simulink model "QAM64_06"  (Simulink 6.6)
settings: Solver=VariableStepDiscrete  StartTime=0.0  StopTime=64*1024/112e6  RelTol=1e-3
undefined symbols (not defined in the file): get, xlfda_numerator
libraries: xbsIndex_r4 x20, dspsnks4 x4, dspsigops x2
settings Model: Creator=lcrockett  LastModifiedBy=lcrockett
settings OptimizationCC: InlineParams=on  InlineInvariantSignals=on
settings DebuggingCC: SignalResolutionControl=TryResolveAllWithWarning  MultiTaskDSMMsg=warning  MultiTaskCondExecSysMsg=none  StrictBusMsg=None
settings RTWCC: IncludeERTFirstTime=on

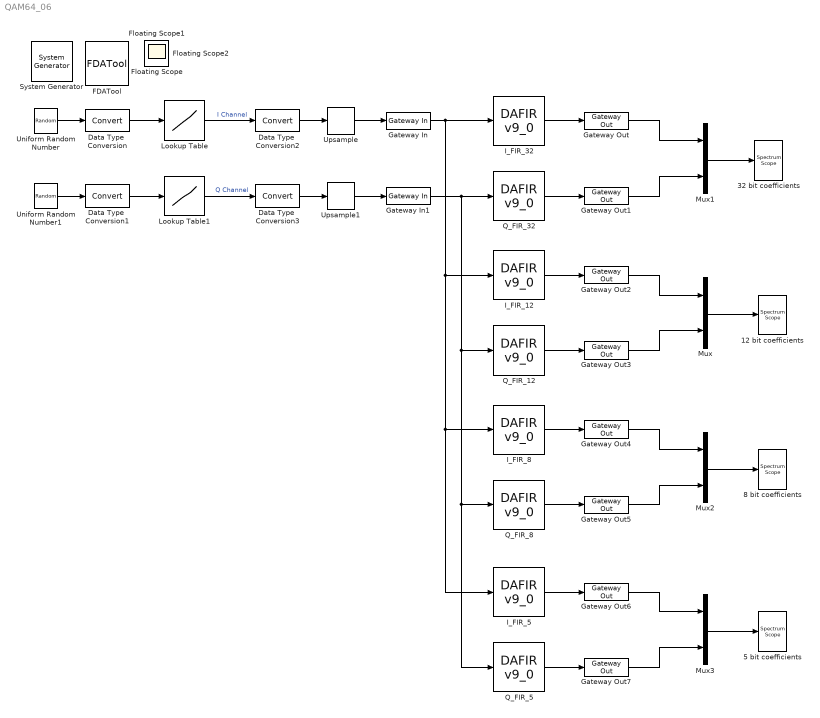
== system QAM64_06 ==
  " System Generator" : xbsIndex_r4/ System Generator  Tag=genX  SystemSampleTime=-1  xilinxfamily=Virtex2  part=xc2v1000  speed=-4  package=bg575  synthesis_tool=XST  directory=./netlist  testbench=off  simulink_period=1/112e6  sysclk_period=100  incr_netlist=off  trim_vbits=Everywhere in SubSystem  dbl_ovrd=According to Block Masks  core_generation=According to Block Masks  run_coregen=off  deprecated_control=off  eval_field=0  block_type=sysgen
      settings: block_version=9.2.01
  12 bit coefficients : dspsnks4/Spectrum Scope  DialogController=dspdialog.SpectrumScope  DialogControllerArgs=DataTag1  SystemSampleTime=-1  ScopeProperties=on  Domain=Frequency  HorizSpan=1  UseBuffer=on  BufferSize=1024  Overlap=64  inpFftLenInherit=on  FFTlength=1024  numAvg=2  DisplayProperties=off  AxisGrid=on  Memory=off  FrameNumber=on  AxisLegend=off  AxisZoom=off  OpenScopeAtSimStart=on  OpenScopeImmediately=off  FigPos=get(0,'defaultfigureposition')  AxisProperties=off  XUnits=Hertz  XRange=[0...Fs/2]  InheritXIncr=off  XIncr=1/112e6  XLabel=Samples  XLimit=Auto  YUnits=dB  XMax=1  XMin=0  YLabel=Magnitude, dB  LineProperties=off  LineColors=[1 0 0]|[0 0 1]  wintypeSpecScope=Hann  RsSpecScope=50  betaSpecScope=5  winsampSpecScope=Periodic
      settings: YMin=-70.9421156820398  YMax=37.379435684992
  32 bit coefficients : dspsnks4/Spectrum Scope  DialogController=dspdialog.SpectrumScope  DialogControllerArgs=DataTag2  SystemSampleTime=-1  ScopeProperties=on  Domain=Frequency  HorizSpan=1  UseBuffer=on  BufferSize=1024  Overlap=64  inpFftLenInherit=on  FFTlength=1024  numAvg=2  DisplayProperties=off  AxisGrid=on  Memory=off  FrameNumber=on  AxisLegend=off  AxisZoom=off  OpenScopeAtSimStart=on  OpenScopeImmediately=off  FigPos=get(0,'defaultfigureposition')  AxisProperties=off  XUnits=Hertz  XRange=[0...Fs/2]  InheritXIncr=off  XIncr=1/112e6  XLabel=Samples  XLimit=Auto  YUnits=dB  XMax=1  XMin=0  YLabel=Magnitude, dB  LineProperties=off  LineColors=[1 0 0]|[0 0 1]  wintypeSpecScope=Hann  RsSpecScope=50  betaSpecScope=5  winsampSpecScope=Periodic
      settings: YMin=-70.9421156820398  YMax=37.379435684992
  5 bit coefficients : dspsnks4/Spectrum Scope  DialogController=dspdialog.SpectrumScope  DialogControllerArgs=DataTag3  SystemSampleTime=-1  ScopeProperties=on  Domain=Frequency  HorizSpan=1  UseBuffer=on  BufferSize=1024  Overlap=64  inpFftLenInherit=on  FFTlength=1024  numAvg=2  DisplayProperties=off  AxisGrid=on  Memory=off  FrameNumber=on  AxisLegend=off  AxisZoom=off  OpenScopeAtSimStart=on  OpenScopeImmediately=off  FigPos=get(0,'defaultfigureposition')  AxisProperties=off  XUnits=Hertz  XRange=[0...Fs/2]  InheritXIncr=off  XIncr=1/112e6  XLabel=Samples  XLimit=Auto  YUnits=dB  XMax=1  XMin=0  YLabel=Magnitude, dB  LineProperties=off  LineColors=[1 0 0]|[0 0 1]  wintypeSpecScope=Hann  RsSpecScope=50  betaSpecScope=5  winsampSpecScope=Periodic
      settings: YMin=-70.9421156820398  YMax=37.379435684992
  8 bit coefficients : dspsnks4/Spectrum Scope  DialogController=dspdialog.SpectrumScope  DialogControllerArgs=DataTag4  SystemSampleTime=-1  ScopeProperties=on  Domain=Frequency  HorizSpan=1  UseBuffer=on  BufferSize=1024  Overlap=64  inpFftLenInherit=on  FFTlength=1024  numAvg=2  DisplayProperties=off  AxisGrid=on  Memory=off  FrameNumber=on  AxisLegend=off  AxisZoom=off  OpenScopeAtSimStart=on  OpenScopeImmediately=off  FigPos=get(0,'defaultfigureposition')  AxisProperties=off  XUnits=Hertz  XRange=[0...Fs/2]  InheritXIncr=off  XIncr=1/112e6  XLabel=Samples  XLimit=Auto  YUnits=dB  XMax=1  XMin=0  YLabel=Magnitude, dB  LineProperties=off  LineColors=[1 0 0]|[0 0 1]  wintypeSpecScope=Hann  RsSpecScope=50  betaSpecScope=5  winsampSpecScope=Periodic
      settings: YMin=-70.9421156820398  YMax=37.379435684992
  Data Type  Conversion : DataTypeConversion  OutDataTypeMode=Specify via dialog  OutDataType=uint(3)  RndMeth=Nearest  SaturateOnIntegerOverflow=on
  Data Type  Conversion1 : DataTypeConversion  OutDataTypeMode=Specify via dialog  OutDataType=uint(3)  RndMeth=Nearest  SaturateOnIntegerOverflow=on
  Data Type  Conversion2 : DataTypeConversion  OutDataTypeMode=Specify via dialog  OutDataType=sfix(8)  SaturateOnIntegerOverflow=on  RndMeth=Zero
  Data Type  Conversion3 : DataTypeConversion  OutDataTypeMode=Specify via dialog  OutDataType=sfix(8)  SaturateOnIntegerOverflow=on  RndMeth=Zero
  FDATool : xbsIndex_r4/FDATool  block_type=fdatool
      settings: infoedit=FDATool  block_version=9.2.01
  Gateway In : xbsIndex_r4/Gateway In  arith_type="Signed  (2's comp)"  n_bits=8  bin_pt=0  quantization=Truncate  overflow=Wrap  period=1/112e6  dbl_ovrd=off  timing_constraint=None  locs_specified=off  LOCs={}  block_type=gatewayin
      settings: infoedit="Gateway in block.  Converts inputs of type Simulink integer, double and fixed point to  Xilinx fixed point type.<P><P>Hardware notes:  In hardware these blocks become top level input ports."  xl_area=[0, 0, 0, 0, 0, 0, 0]  block_version=VER_STRING_GOES_HERE
  Gateway In1 : xbsIndex_r4/Gateway In  arith_type="Signed  (2's comp)"  n_bits=8  bin_pt=0  quantization=Truncate  overflow=Wrap  period=1/112e6  dbl_ovrd=off  timing_constraint=None  locs_specified=off  LOCs={}  block_type=gatewayin
      settings: infoedit="Gateway in block.  Converts inputs of type Simulink integer, double and fixed point to  Xilinx fixed point type.<P><P>Hardware notes:  In hardware these blocks become top level input ports."  xl_area=[0, 0, 0, 0, 0, 0, 0]  block_version=VER_STRING_GOES_HERE
  Gateway Out{,1..7} (8 alike) : xbsIndex_r4/Gateway Out  hdl_port=off  timing_constraint=None  locs_specified=off  LOCs={}  block_type=gatewayout
      settings: infoedit="Gateway out block.  Converts Xilinx fixed point inputs into ouputs of type Simulink integer, double, or fixed point.<P><P>Hardware notes:  In hardware these blocks become top level output ports or are discarded, depending on how they are configured."  xl_area=[0, 0, 0, 0, 0, 0, 0]  block_version=VER_STRING_GOES_HERE
  I_FIR_12 : xbsIndex_r4/DAFIR v9_0   coef=xlfda_numerator('FDATool')  structure=Inferred from Coefficients  coef_n_bits=12  coef_bin_pt=11  over_sample=1  reload=off  valids=off  rst=off  latency=1  num_channels=1  serial_input=off  polyphase_behavior="Single Rate:  sample in - sample out"  dbl_ovrd=off  explicit_period=off  period=1  use_isim=0  block_type=fir
      settings: infoedit="Hardware notes: Implemented using distributed arithmetic (DA).  The hardware over sampling rate determines the degree of parallelism.  A rate of one produces a fully parallel DA filter.  A rate of n (resp., n+1) for an n-bit input signal produces a fully serial implementation for a non-symmetric (resp., symmetric) impulse response.  Intermediate values produce implementations with intermediate levels of parallelism."  xl_area=[0, 0, 0, 0, 0, 0, 0]  block_version=VER_STRING_GOES_HERE
  I_FIR_32 : xbsIndex_r4/DAFIR v9_0   coef=xlfda_numerator('FDATool')  structure=Inferred from Coefficients  coef_n_bits=32  coef_bin_pt=31  over_sample=1  reload=off  valids=off  rst=off  latency=1  num_channels=1  serial_input=off  polyphase_behavior="Single Rate:  sample in - sample out"  dbl_ovrd=on  explicit_period=off  period=1  use_isim=0  block_type=fir
      settings: infoedit="Hardware notes: Implemented using distributed arithmetic (DA).  The hardware over sampling rate determines the degree of parallelism.  A rate of one produces a fully parallel DA filter.  A rate of n (resp., n+1) for an n-bit input signal produces a fully serial implementation for a non-symmetric (resp., symmetric) impulse response.  Intermediate values produce implementations with intermediate levels of parallelism."  xl_area=[0, 0, 0, 0, 0, 0, 0]  block_version=VER_STRING_GOES_HERE
  I_FIR_5 : xbsIndex_r4/DAFIR v9_0   coef=xlfda_numerator('FDATool')  structure=Inferred from Coefficients  coef_n_bits=5  coef_bin_pt=4  over_sample=1  reload=off  valids=off  rst=off  latency=1  num_channels=1  serial_input=off  polyphase_behavior="Single Rate:  sample in - sample out"  dbl_ovrd=off  explicit_period=off  period=1  use_isim=0  block_type=fir
      settings: infoedit="Hardware notes: Implemented using distributed arithmetic (DA).  The hardware over sampling rate determines the degree of parallelism.  A rate of one produces a fully parallel DA filter.  A rate of n (resp., n+1) for an n-bit input signal produces a fully serial implementation for a non-symmetric (resp., symmetric) impulse response.  Intermediate values produce implementations with intermediate levels of parallelism."  xl_area=[0, 0, 0, 0, 0, 0, 0]  block_version=VER_STRING_GOES_HERE
  I_FIR_8 : xbsIndex_r4/DAFIR v9_0   coef=xlfda_numerator('FDATool')  structure=Inferred from Coefficients  coef_n_bits=8  coef_bin_pt=7  over_sample=1  reload=off  valids=off  rst=off  latency=1  num_channels=1  serial_input=off  polyphase_behavior="Single Rate:  sample in - sample out"  dbl_ovrd=off  explicit_period=off  period=1  use_isim=0  block_type=fir
      settings: infoedit="Hardware notes: Implemented using distributed arithmetic (DA).  The hardware over sampling rate determines the degree of parallelism.  A rate of one produces a fully parallel DA filter.  A rate of n (resp., n+1) for an n-bit input signal produces a fully serial implementation for a non-symmetric (resp., symmetric) impulse response.  Intermediate values produce implementations with intermediate levels of parallelism."  xl_area=[0, 0, 0, 0, 0, 0, 0]  block_version=VER_STRING_GOES_HERE
  Lookup Table : Lookup  InputValues=[0 1 2 3 4 5 6 7]  OutputValues=[127 90.71428571 54.42857143 18.14285714 -18.14285714 -54.42857143 -90.71428571 -127]  OutDataTypeMode=Specify via dialog  OutDataType=float('double')
  Lookup Table1 : Lookup  InputValues=[0 1 2 3 4 5 6 7]  OutputValues=[127 90.71428571 54.42857143 18.14285714 -18.14285714 -54.42857143 -90.71428571 -127]  OutDataTypeMode=Specify via dialog  OutDataType=float('double')
  Mux{,1..3} (4 alike) : Mux  Inputs=2
  Q_FIR_12 : xbsIndex_r4/DAFIR v9_0   coef=xlfda_numerator('FDATool')  structure=Inferred from Coefficients  coef_n_bits=12  coef_bin_pt=11  over_sample=1  reload=off  valids=off  rst=off  latency=1  num_channels=1  serial_input=off  polyphase_behavior="Single Rate:  sample in - sample out"  dbl_ovrd=off  explicit_period=off  period=1  use_isim=0  block_type=fir
      settings: infoedit="Hardware notes: Implemented using distributed arithmetic (DA).  The hardware over sampling rate determines the degree of parallelism.  A rate of one produces a fully parallel DA filter.  A rate of n (resp., n+1) for an n-bit input signal produces a fully serial implementation for a non-symmetric (resp., symmetric) impulse response.  Intermediate values produce implementations with intermediate levels of parallelism."  xl_area=[0, 0, 0, 0, 0, 0, 0]  block_version=VER_STRING_GOES_HERE
  Q_FIR_32 : xbsIndex_r4/DAFIR v9_0   coef=xlfda_numerator('FDATool')  structure=Inferred from Coefficients  coef_n_bits=32  coef_bin_pt=31  over_sample=1  reload=off  valids=off  rst=off  latency=1  num_channels=1  serial_input=off  polyphase_behavior="Single Rate:  sample in - sample out"  dbl_ovrd=on  explicit_period=off  period=1  use_isim=0  block_type=fir
      settings: infoedit="Hardware notes: Implemented using distributed arithmetic (DA).  The hardware over sampling rate determines the degree of parallelism.  A rate of one produces a fully parallel DA filter.  A rate of n (resp., n+1) for an n-bit input signal produces a fully serial implementation for a non-symmetric (resp., symmetric) impulse response.  Intermediate values produce implementations with intermediate levels of parallelism."  xl_area=[0, 0, 0, 0, 0, 0, 0]  block_version=VER_STRING_GOES_HERE
  Q_FIR_5 : xbsIndex_r4/DAFIR v9_0   coef=xlfda_numerator('FDATool')  structure=Inferred from Coefficients  coef_n_bits=5  coef_bin_pt=4  over_sample=1  reload=off  valids=off  rst=off  latency=1  num_channels=1  serial_input=off  polyphase_behavior="Single Rate:  sample in - sample out"  dbl_ovrd=off  explicit_period=off  period=1  use_isim=0  block_type=fir
      settings: infoedit="Hardware notes: Implemented using distributed arithmetic (DA).  The hardware over sampling rate determines the degree of parallelism.  A rate of one produces a fully parallel DA filter.  A rate of n (resp., n+1) for an n-bit input signal produces a fully serial implementation for a non-symmetric (resp., symmetric) impulse response.  Intermediate values produce implementations with intermediate levels of parallelism."  xl_area=[0, 0, 0, 0, 0, 0, 0]  block_version=VER_STRING_GOES_HERE
  Q_FIR_8 : xbsIndex_r4/DAFIR v9_0   coef=xlfda_numerator('FDATool')  structure=Inferred from Coefficients  coef_n_bits=8  coef_bin_pt=7  over_sample=1  reload=off  valids=off  rst=off  latency=1  num_channels=1  serial_input=off  polyphase_behavior="Single Rate:  sample in - sample out"  dbl_ovrd=off  explicit_period=off  period=1  use_isim=0  block_type=fir
      settings: infoedit="Hardware notes: Implemented using distributed arithmetic (DA).  The hardware over sampling rate determines the degree of parallelism.  A rate of one produces a fully parallel DA filter.  A rate of n (resp., n+1) for an n-bit input signal produces a fully serial implementation for a non-symmetric (resp., symmetric) impulse response.  Intermediate values produce implementations with intermediate levels of parallelism."  xl_area=[0, 0, 0, 0, 0, 0, 0]  block_version=VER_STRING_GOES_HERE
  Uniform Random Number : UniformRandomNumber  Minimum=0  Maximum=7  SampleTime=1/28e6
  Uniform Random Number1 : UniformRandomNumber  Minimum=0  Maximum=7  Seed=1  SampleTime=1/28e6
  Upsample : dspsigops/Upsample  N=4  phase=0  ic=0  mode=Maintain input frame size
  Upsample1 : dspsigops/Upsample  N=4  phase=0  ic=0  mode=Maintain input frame size
  Floating Scope : Scope
      settings: Floating=on  YMin=-150  YMax=150
  Floating Scope1 : Scope
      settings: Floating=on
  Floating Scope2 : Scope
      settings: Floating=on
  wires:
  Uniform Random Number/1 -> Data Type  Conversion/1
  Data Type  Conversion1/1 -> Lookup Table1/1
  Uniform Random Number1/1 -> Data Type  Conversion1/1
  Data Type  Conversion/1 -> Lookup Table/1
  Lookup Table/1 -> Data Type  Conversion2/1  "I Channel"
  Data Type  Conversion2/1 -> Upsample/1
  Lookup Table1/1 -> Data Type  Conversion3/1  "Q Channel"
  Data Type  Conversion3/1 -> Upsample1/1
  Upsample/1 -> Gateway In/1
  Gateway In/1 -> I_FIR_32/1, I_FIR_12/1, I_FIR_8/1, I_FIR_5/1
  Upsample1/1 -> Gateway In1/1
  Gateway In1/1 -> Q_FIR_32/1, Q_FIR_12/1, Q_FIR_8/1, Q_FIR_5/1
  I_FIR_32/1 -> Gateway Out/1
  Q_FIR_32/1 -> Gateway Out1/1
  I_FIR_12/1 -> Gateway Out2/1
  Q_FIR_12/1 -> Gateway Out3/1
  I_FIR_8/1 -> Gateway Out4/1
  Q_FIR_8/1 -> Gateway Out5/1
  I_FIR_5/1 -> Gateway Out6/1
  Q_FIR_5/1 -> Gateway Out7/1
  Mux2/1 -> 8 bit coefficients/1
  Mux/1 -> 12 bit coefficients/1
  Mux1/1 -> 32 bit coefficients/1
  Gateway Out/1 -> Mux1/1
  Gateway Out1/1 -> Mux1/2
  Gateway Out2/1 -> Mux/1
  Gateway Out3/1 -> Mux/2
  Gateway Out4/1 -> Mux2/1
  Gateway Out5/1 -> Mux2/2
  Mux3/1 -> 5 bit coefficients/1
  Gateway Out6/1 -> Mux3/1
  Gateway Out7/1 -> Mux3/2
